simulink model "VendingMachine"  (R2020a)
settings: Solver=VariableStepAuto  StartTime=0.0  StopTime=1500  RelTol=1e-3
settings Model: EnablePacing=on  PacingRate=10  Creator=jatin  LastModifiedBy=jatin
settings SolverCC: AlgebraicLoopSolver=LineSearch

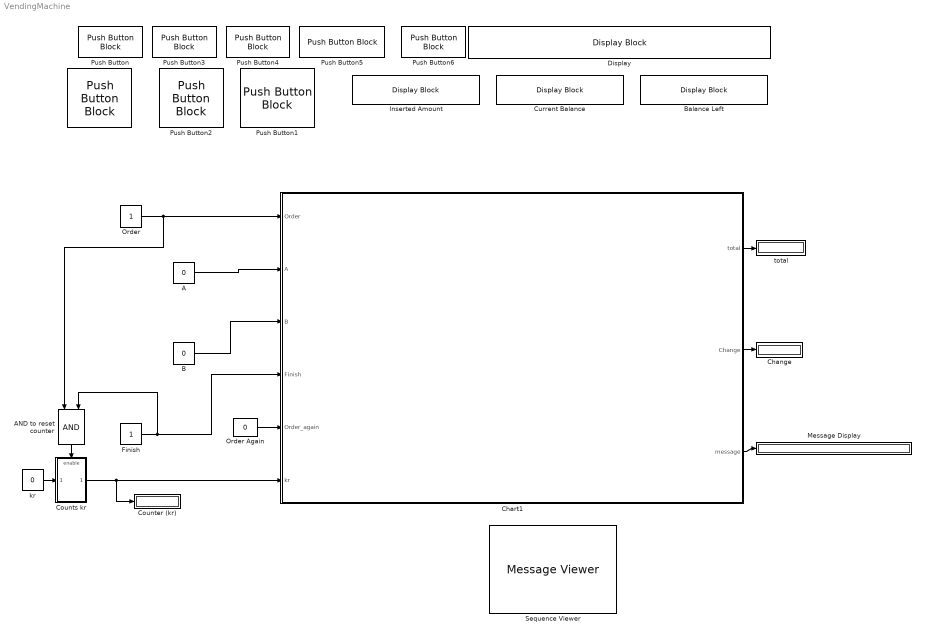
== system VendingMachine ==
  " " : PushButtonBlock  ButtonText=1kr
  A : Constant  Value=0
  AND to reset counter : Logic  IconShape=distinctive  AllPortsSameDT=off  OutDataTypeStr=boolean
  B : Constant  Value=0
  Balance Left : DisplayBlock  LabelPosition=Hide  Format=short  Transparency=1
  Change : Display
  Chart1 : Stateflow chart  TreatAsAtomicUnit=on
  Counter (kr) : Display
  Counts kr : Subsystem
  Current Balance : DisplayBlock  LabelPosition=Hide  Format=short  Transparency=1
  Display : DisplayBlock  LabelPosition=Hide  Format=short  Transparency=1
  Finish : Constant
  Inserted Amount : DisplayBlock  LabelPosition=Hide  Format=short  Transparency=1
  Message Display : Display
  Order : Constant
  Order Again : Constant  Value=0
  Push Button : PushButtonBlock  ButtonText=Order  OnValue=0
  Push Button1 : PushButtonBlock  ButtonText=10kr  OnValue=10
  Push Button2 : PushButtonBlock  ButtonText=5kr  OnValue=5
  Push Button3 : PushButtonBlock  ButtonText=A  OnValue=100
  Push Button4 : PushButtonBlock  ButtonText=B  OnValue=100
  Push Button5 : PushButtonBlock  ButtonText=Order_again
  Push Button6 : PushButtonBlock  ButtonText=Finish  OnValue=0
  Sequence Viewer : MessageViewer  History=1000  SavedRootId=#
  kr : Constant  Value=0
  total : Display
  wires:
  Order Again/1 -> Chart1/5(Order_again)
  B/1 -> Chart1/3(B)
  Order/1 -> AND to reset counter/1, Chart1/1(Order)
  A/1 -> Chart1/2(A)
  kr/1 -> Counts kr/1(In1)
  Counts kr/1(Out1) -> Counter (kr)/1, Chart1/6(kr)
  Finish/1 -> AND to reset counter/2, Chart1/4(Finish)
  AND to reset counter/1 -> Counts kr/Enable
  Chart1/1(total) -> total/1
  Chart1/2(Change) -> Change/1
  Chart1/3(message) -> Message Display/1

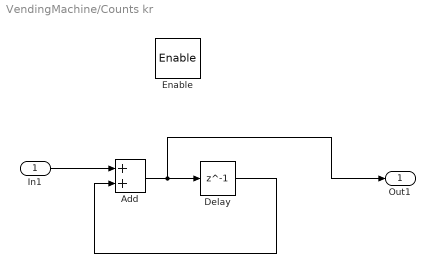
== system VendingMachine/Counts kr ==
  In1 : Inport
  Enable : EnablePort  StatesWhenEnabling=reset
  Add : Sum
  Delay : Delay  DelayLength=1
  Out1 : Outport
  wires:
  Add/1 -> Out1/1, Delay/1
  In1/1 -> Add/1
  Delay/1 -> Add/2

== stateflow chart VendingMachine/Chart1 ==
  settings: executeAtInitialization=1
  state CalChangeA
    Change = total-8;
    message = "Finish to collect change or Order more snacks";
  state A
    message = "A selected";
  state IdleState
    en: coins=0; Change=0; total=0;
    message = "Welcome! Insert coins";
  state InsertingState
    du: coins = kr;
    message = "Insert coins and press order";
    ex: total = total + coins;
  state OrdAgain
    total=Change;
  state OrderState
    message="Select A or B";
  state CalChangeB
    Change = total-6;
    message = "Finish to collect change or order more snacks";
  state B
    message = "B selected";
  CalChangeA -> IdleState [order 1] : [Finish<1]{message = "Collect Balance";}
  A -> InsertingState [order 1] : [total<8]{message = "Sorry! Low Balance";}
  InsertingState -> IdleState [order 2] : [Finish<1]{message="Collect Balance";}
  (default) -> IdleState
  A -> CalChangeA [order 2] : [total>=8]
  CalChangeA -> OrdAgain [order 2] : [Order_again>0]
  OrderState -> A [order 1] : [A>0]
  IdleState -> InsertingState : [kr>0]
  CalChangeB -> OrdAgain [order 1] : [Order_again>0]
  InsertingState -> OrderState [order 1] : [Order<1]
  OrderState -> B [order 2] : [B>0]
  OrdAgain -> InsertingState [order 2] : [total<=0]
  OrdAgain -> OrderState [order 1] : [total>0]
  B -> CalChangeB [order 2] : [total>=6]
  B -> InsertingState [order 1] : [total<6]{message = "Sorry! Low Balance";}
  CalChangeB -> IdleState [order 2] : [Finish<1]/{message="Collect Balance";}
  data: Order input; A input; B input; Finish input; Order_again input; kr input; coins local double; total output double; Change output double; message output string
